simulink model "HW2_FSR_ES2"  (R2023b)
settings: Solver=ode23  StartTime=0.0  StopTime=T+1  FixedStep=0.001  RelTol=1e-5
values from neighbouring files (symbols this model uses):
  b = 0.6    [HW2_FSR_ES1_ES2_Script.m]
  dt = 0.001    [HW2_FSR_ES1_ES2_Script.m]
  k_1 = 60    [HW2_FSR_ES1_ES2_Script.m]
libraries: robotmobilelib x1
settings Model: Creator=emman  LastModifiedBy=emman

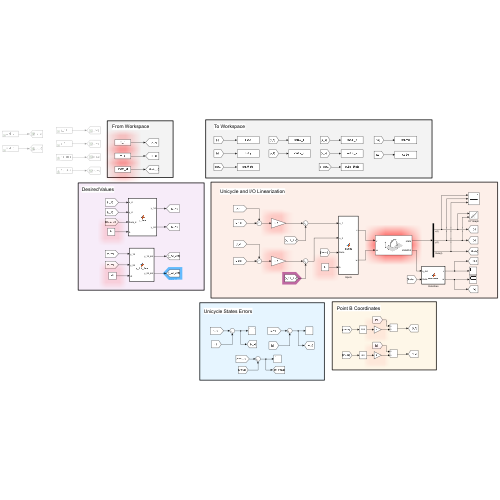
[thumbnail: Simulink's stored preview of the top-level diagram]
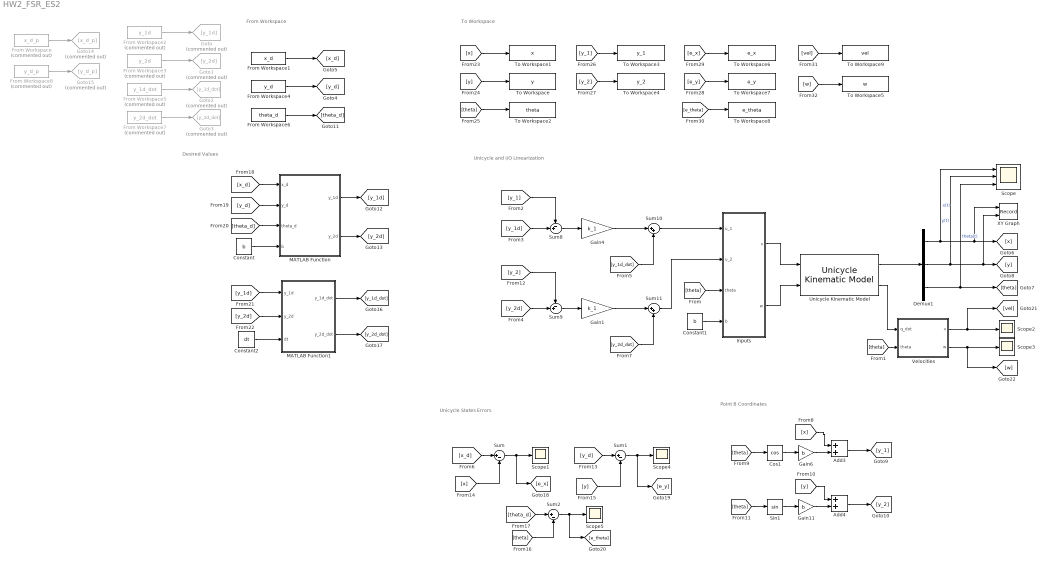
== system HW2_FSR_ES2 ==
  note: Desired Values
  note: Unicycle and I/O Linearization
  note: From Workspace
  note: Point B Coordinates
  note: Unicycle States Errors
  note: To Workspace
  Add3 : Sum
  Add4 : Sum
  Constant : Constant  Value=b
  Constant1 : Constant  Value=b
  Constant2 : Constant  Value=dt
  Cos1 : Trigonometry  Operator=cos
  Demux1 : Demux  Outputs=3
  From Workspace : FromWorkspace  Commented=on  VariableName=x_d_p
  From Workspace1 : FromWorkspace  VariableName=x_d  OutputAfterFinalValue=Holding final value
  From Workspace2 : FromWorkspace  Commented=on  VariableName=y_1d  OutputAfterFinalValue=Holding final value
  From Workspace3 : FromWorkspace  Commented=on  VariableName=y_2d  OutputAfterFinalValue=Holding final value
  From Workspace4 : FromWorkspace  VariableName=y_d  OutputAfterFinalValue=Holding final value
  From Workspace5 : FromWorkspace  Commented=on  VariableName=y_1d_dot  OutputAfterFinalValue=Holding final value
  From Workspace6 : FromWorkspace  VariableName=theta_d  OutputAfterFinalValue=Holding final value
  From Workspace7 : FromWorkspace  Commented=on  VariableName=y_2d_dot  OutputAfterFinalValue=Holding final value
  From Workspace8 : FromWorkspace  Commented=on  VariableName=y_d_p
  Gain1 : Gain  Gain=k_1
  Gain11 : Gain  Gain=b
  Gain4 : Gain  Gain=k_1
  Gain6 : Gain  Gain=b
  Goto : Goto  Commented=on  GotoTag=y_1d
  Goto1 : Goto  Commented=on  GotoTag=y_2d
  Goto14 : Goto  Commented=on  GotoTag=x_d_p
  Goto15 : Goto  Commented=on  GotoTag=y_d_p
  Goto2 : Goto  Commented=on  GotoTag=y_1d_dot
  Goto3 : Goto  Commented=on  GotoTag=y_2d_dot
  Inputs : MATLAB Function  TreatAsAtomicUnit=on
  MATLAB Function : MATLAB Function  TreatAsAtomicUnit=on
  MATLAB Function1 : MATLAB Function  TreatAsAtomicUnit=on
  Scope : Scope  NumInputPorts=3
  Scope{1..5} (5 alike) : Scope
  Sin1 : Trigonometry
  Sum : Sum  Inputs=|+-
  Sum1 : Sum  Inputs=|+-
  Sum10 : Sum  Inputs=|++
  Sum11 : Sum  Inputs=|++
  Sum2 : Sum  Inputs=|+-
  Sum8 : Sum  Inputs=-+|
  Sum9 : Sum  Inputs=-+|
  To Workspace : ToWorkspace  VariableName=y  SaveFormat=Timeseries  SampleTime=-1
  To Workspace1 : ToWorkspace  VariableName=x  SaveFormat=Timeseries  SampleTime=-1
  To Workspace2 : ToWorkspace  VariableName=theta  SaveFormat=Timeseries  SampleTime=-1
  To Workspace3 : ToWorkspace  VariableName=y_1  SaveFormat=Timeseries  SampleTime=-1
  To Workspace4 : ToWorkspace  VariableName=y_2  SaveFormat=Timeseries  SampleTime=-1
  To Workspace5 : ToWorkspace  VariableName=w  SaveFormat=Timeseries  SampleTime=-1
  To Workspace6 : ToWorkspace  VariableName=e_x  SaveFormat=Timeseries  SampleTime=-1
  To Workspace7 : ToWorkspace  VariableName=e_y  SaveFormat=Timeseries  SampleTime=-1
  To Workspace8 : ToWorkspace  VariableName=e_theta  SaveFormat=Timeseries  SampleTime=-1
  To Workspace9 : ToWorkspace  VariableName=vel  SaveFormat=Timeseries  SampleTime=-1
  Unicycle Kinematic Model : robotmobilelib/Unicycle Kinematic Model  VehicleInputs=Vehicle Speed & Heading Angular Velocity  WheelRadius=0.1  WheelSpeedRange=[-Inf Inf]  InitialState=q_i  SimulateUsing=Interpreted execution
  Velocities : MATLAB Function  TreatAsAtomicUnit=on
  XY Graph : Record  FileSettingsInternal="{\"entries\":[{\"content\":{\"excelSettings\":{\"content\":{},\"type\":\"Streamout.ExcelSettings\"}},\"type\":\"Streamout.FileSettingStorage\",\"uuid\":\"\"}],\"packageUris\":[\"http:\\/\\/schema.mathworks.com\\/mf0\\/streamout_blocks\\/R2020a\"],\"version\":\"1.0\"}"  Layout=[1 1]  SignalsInternal="{\"entries\":[{\"content\":{\"signals\":[{\"content\":{\"blockPath\":[],\"dimensions\":[1],\"domain\":\"\",\"lineColor\":\"#a2142f\",\"plots\":[1],\"port\":1,\"signalID\":8,\"signalName\":\"x(t)\"},\"type\":\"RecordBlkView.Signal\",\"uuid\":\"\"},{\"content\":{\"blockPath\":[],\"dimensions\":[1],\"domain\":\"\",\"lineColor\":\"#139fff\",\"plots\":[1],\"port\":2,\"signalID\":11,\"signalName\":\"y(t)\"},\"type\":\"RecordBlkView.Signal\",\"uuid\":\"\"}]},\"type\":\"RecordBlkView.InputSignals\",\"uuid\":\"\"}],\"packageUris\":[\"http:\\/\\/schema.mathworks.com\\/mf0\\/streamout_blocks\\/R2020a\"],\"version\":\"1.0\"}"  VisualizationBindings="{\"xyplotplugin\":{\"info\":[{\"series\":[{\"bindingParametersList\":[{\"parameter\":\"X-Axis\",\"signalID\":8,\"signalName\":\"x(t)\"},{\"parameter\":\"Y-Axis\",\"signalID\":11,\"signalName\":\"y(t)\"}],\"seriesID\":48537}],\"subplotID\":1}]}}"  CompatibilityTag=XY
  wires:
  [y_1] -> Sum8/1
  [y_2] -> Sum9/1
  Sum8/1 -> Gain4/1
  Gain4/1 -> Sum10/1
  [y_1d_dot] -> Sum10/2
  [y_2d_dot] -> Sum11/2
  Constant1/1 -> Inputs/4(b)
  Sum11/1 -> Inputs/2(u_2)
  Sum10/1 -> Inputs/1(u_1)
  Inputs/1(v) -> Unicycle Kinematic Model/1
  Inputs/2(w) -> Unicycle Kinematic Model/2
  [x] -> Add3/1
  [y] -> Add4/1
  Demux1/1 -> Scope/1, [x], XY Graph/1  "x(t)"
  Demux1/3 -> Scope/3, [theta]  "theta(t)"
  Gain11/1 -> Add4/2
  Add3/1 -> [y_1]
  Sin1/1 -> Gain11/1
  Demux1/2 -> Scope/2, [y], XY Graph/2  "y(t)"
  Cos1/1 -> Gain6/1
  Gain6/1 -> Add3/2
  [theta] -> Sin1/1
  [theta] -> Cos1/1
  Add4/1 -> [y_2]
  Unicycle Kinematic Model/1 -> Demux1/1
  [theta] -> Inputs/3(theta)
  [y_2d] -> Sum9/2
  Velocities/1(v) -> Scope2/1, [vel]
  Velocities/2(w) -> Scope3/1, [w]
  Unicycle Kinematic Model/2 -> Velocities/1(q_dot)
  [theta] -> Velocities/2(theta)
  From Workspace7/1 -> Goto3/1
  From Workspace5/1 -> Goto2/1
  From Workspace3/1 -> Goto1/1
  From Workspace2/1 -> Goto/1
  [y_1d] -> Sum8/2
  Sum9/1 -> Gain1/1
  Gain1/1 -> Sum11/1
  From Workspace1/1 -> [x_d]
  From Workspace4/1 -> [y_d]
  [x_d] -> Sum/1
  [x] -> Sum/2
  [y_d] -> Sum1/1
  [y] -> Sum1/2
  Sum1/1 -> [e_y], Scope4/1
  Sum/1 -> [e_x], Scope1/1
  From Workspace6/1 -> [theta_d]
  Sum2/1 -> [e_theta], Scope5/1
  [theta] -> Sum2/2
  [theta_d] -> Sum2/1
  [theta_d] -> MATLAB Function/3(theta_d)
  [y_d] -> MATLAB Function/2(y_d)
  [x_d] -> MATLAB Function/1(x_d)
  Constant/1 -> MATLAB Function/4(b)
  MATLAB Function/1(y_1d) -> [y_1d]
  MATLAB Function/2(y_2d) -> [y_2d]
  From Workspace/1 -> Goto14/1
  From Workspace8/1 -> Goto15/1
  [y_1d] -> MATLAB Function1/1(y_1d)
  [y_2d] -> MATLAB Function1/2(y_2d)
  Constant2/1 -> MATLAB Function1/3(dt)
  MATLAB Function1/1(y_1d_dot) -> [y_1d_dot]
  MATLAB Function1/2(y_2d_dot) -> [y_2d_dot]
  [x] -> To Workspace1/1
  [y] -> To Workspace/1
  [theta] -> To Workspace2/1
  [y_1] -> To Workspace3/1
  [y_2] -> To Workspace4/1
  [e_y] -> To Workspace7/1
  [e_x] -> To Workspace6/1
  [e_theta] -> To Workspace8/1
  [vel] -> To Workspace9/1
  [w] -> To Workspace5/1

== matlab function HW2_FSR_ES2/Inputs ==
  data: u_1 input; u_2 input; theta input; b input; v output; w output
function [v,w] = inputs(u_1, u_2, theta, b)

T = [cos(theta) -b*sin(theta);
     sin(theta) b*cos(theta)];

Tinv = inv(T);

% v = Tinv(1,1)*u_1+Tinv(1,2)*u_2;
% w = Tinv(2,1)*u_1+Tinv(2,2)*u_2;

vel = Tinv*[u_1;u_2];

v = vel(1);
w = vel(2);

== matlab function HW2_FSR_ES2/Velocities ==
  data: q_dot input; v output; w output; theta input
function [v,w] = velocities(q_dot, theta)

v= q_dot(1)/cos(theta);
w= q_dot(3);

== matlab function HW2_FSR_ES2/MATLAB Function ==
  data: x_d input; y_1d output; y_d input; theta_d input; b input; y_2d output
function [y_1d,y_2d] = y_des(x_d, y_d, theta_d, b)

y_1d = x_d + b.*cos(theta_d);
y_2d = y_d + b.*sin(theta_d);

== matlab function HW2_FSR_ES2/MATLAB Function1 ==
  data: y_1d input; y_1d_dot output; y_2d input; dt input; y_2d_dot output
function [y_1d_dot, y_2d_dot]  = y_dot_des(y_1d, y_2d, dt)

y_1d_dot = gradient(y_1d, dt);
y_2d_dot = gradient(y_2d, dt);
